simulink model "Uklad_simulink_vivado_trzy_sciezki_works"  (R2025b)
settings: Solver=VariableStepAuto  StartTime=0.0  StopTime=0.5  RelTol=1e-3
undefined symbols (not defined in the file or in its folder): c, dspblkCoreblockFVToolHelper, gcbh, sfvc784, xck26
libraries: hdlBasic x7, simulink x4, hdlDSPIP x3, hdlUtilities x2, vmcUtilities x1
settings Model: Creator=janek  LastModifiedBy=janek

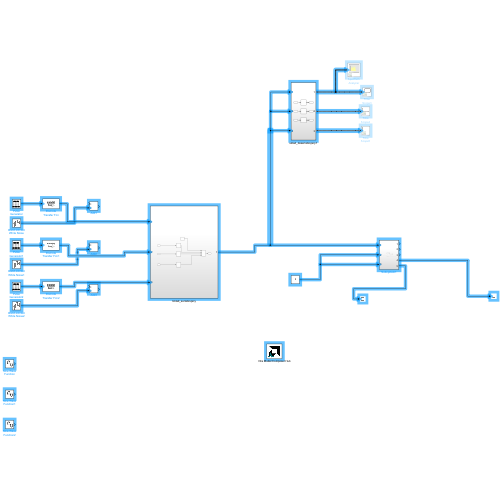
[thumbnail: Simulink's stored preview of the top-level diagram]
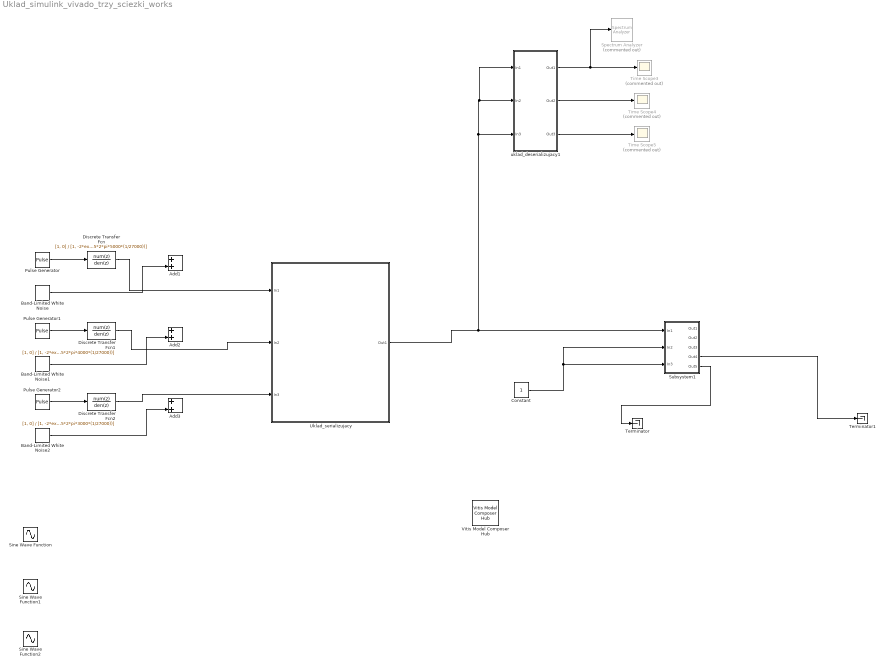
== system Uklad_simulink_vivado_trzy_sciezki_works ==
  Add1 : Sum
  Add2 : Sum
  Add3 : Sum
  Band-Limited White Noise : simulink/Sources/Band-Limited White Noise  Cov=[0.000001]  Ts=1/27000  seed=[23341]
  Band-Limited White Noise1 : simulink/Sources/Band-Limited White Noise  Cov=[0.000005]  Ts=1/27000  seed=[23341]
  Band-Limited White Noise2 : simulink/Sources/Band-Limited White Noise  Cov=[0.000005]  Ts=1/27000  seed=[23341]
  Constant : Constant
  Discrete Transfer Fcn : DiscreteTransferFcn  LoadFcn=dspblkCoreblockFVToolHelper(gcbh,'load');  Numerator=[1, 0]  Denominator=[1, -2*exp(-0.05*2*pi*5000*(1/27000))*cos(2*pi*5000*sqrt(1-0.05^2)*(1/27000)), exp(-2*0.05*2*pi*5000*(1/27000))]
      settings: CopyFcn=dspblkCoreblockFVToolHelper(gcbh,'copy');  DeleteFcn=dspblkCoreblockFVToolHelper(gcbh,'close');  ModelCloseFcn=dspblkCoreblockFVToolHelper(gcbh,'close');  PreSaveFcn=dspblkCoreblockFVToolHelper(gcbh,'presave');  PostSaveFcn=dspblkCoreblockFVToolHelper(gcbh,'postsave');  CloseFcn=dspblkCoreblockFVToolHelper(gcbh,'close');
  Discrete Transfer Fcn1 : DiscreteTransferFcn  LoadFcn=dspblkCoreblockFVToolHelper(gcbh,'load');  Numerator=[1, 0]  Denominator=[1, -2*exp(-0.05*2*pi*5000*(1/27000))*cos(2*pi*4000*sqrt(1-0.05^2)*(1/27000)), exp(-2*0.05*2*pi*4000*(1/27000))]
      settings: CopyFcn=dspblkCoreblockFVToolHelper(gcbh,'copy');  DeleteFcn=dspblkCoreblockFVToolHelper(gcbh,'close');  ModelCloseFcn=dspblkCoreblockFVToolHelper(gcbh,'close');  PreSaveFcn=dspblkCoreblockFVToolHelper(gcbh,'presave');  PostSaveFcn=dspblkCoreblockFVToolHelper(gcbh,'postsave');  CloseFcn=dspblkCoreblockFVToolHelper(gcbh,'close');
  Discrete Transfer Fcn2 : DiscreteTransferFcn  LoadFcn=dspblkCoreblockFVToolHelper(gcbh,'load');  Numerator=[1, 0]  Denominator=[1, -2*exp(-0.05*2*pi*5000*(1/27000))*cos(2*pi*3000*sqrt(1-0.05^2)*(1/27000)), exp(-2*0.05*2*pi*3000*(1/27000))]
      settings: CopyFcn=dspblkCoreblockFVToolHelper(gcbh,'copy');  DeleteFcn=dspblkCoreblockFVToolHelper(gcbh,'close');  ModelCloseFcn=dspblkCoreblockFVToolHelper(gcbh,'close');  PreSaveFcn=dspblkCoreblockFVToolHelper(gcbh,'presave');  PostSaveFcn=dspblkCoreblockFVToolHelper(gcbh,'postsave');  CloseFcn=dspblkCoreblockFVToolHelper(gcbh,'close');
  Pulse Generator : DiscretePulseGenerator  Period=540  SampleTime=1/27000
  Pulse Generator1 : DiscretePulseGenerator  Period=675  SampleTime=1/27000
  Pulse Generator2 : DiscretePulseGenerator  Period=900  SampleTime=1/27000
  Sine Wave Function : Sin  Frequency=2*pi*4000  SampleTime=1/27000
  Sine Wave Function1 : Sin  Frequency=2*pi*5000  SampleTime=1/27000
  Sine Wave Function2 : Sin  Frequency=2*pi*3000  SampleTime=1/27000
  Spectrum Analyzer : SpectrumAnalyzer  Commented=on  WindowPosition=[727.000000,50.000000,800.000000,510.000000,]  ScopeFrameLocation=window  SampleRateSource=Property  SampleRate=27000  WindowInvariantSamplesPerUpdate=on  Span=27000  StartFrequency=-13500  StopFrequency=13500  YLimits=[-62.2796 1.3485]  SelectedToolstripTab=spectrumAnalyzerToolstrip.measurementsTab
  Subsystem1 : Subsystem
  Terminator : Terminator
  Terminator1 : Terminator
  Time Scope3 : Scope  Commented=on
      settings: TimeUnits=Metric (based on Time Span)  ActiveDisplayYMinimum=-1.152524294390888  ActiveDisplayYMaximum=1.239169366043442  YLabel=Amplitude  DataLoggingVariableName=ScopeData6
  Time Scope4 : Scope  Commented=on
      settings: TimeUnits=Metric (based on Time Span)  ActiveDisplayYMinimum=-1.2987208316479313  ActiveDisplayYMaximum=1.398278565602173  YLabel=Amplitude  DataLoggingVariableName=ScopeData7
  Time Scope5 : Scope  Commented=on
      settings: TimeUnits=Metric (based on Time Span)  ActiveDisplayYMinimum=-1.5119749451959528  ActiveDisplayYMaximum=1.7752831879003923  YLabel=Amplitude  DataLoggingVariableName=ScopeData8
  Uklad_serializujacy : Subsystem
  Vitis Model Composer Hub : vmcUtilities/Vitis Model Composer Hub  Tag=genX  CodeGeneration=off  SubsystemName=Subsystem1  CompilationType=HDLCompilation  ExportTypeV2=IP Catalog  StartColumn=1  NumberOfColumns=1  TargetDirectory=./netlist  exportDesign=off  analyzeDesign=off  validateDesignOnHw=off  ExportType=AI Engines  IpVendor=xilinx.com  IpLibrary=hls  IpVersion=1.0  IpHWLanguage=Verilog  AieCompilerOptions={}  AieSimulatorOptions={}  CreateTestbench=off  TestbenchStackSize=10  RunRtlSim=off  RunCSim=off  RunAieSim=off  AieSimTimeout=50000  RunAieSimProfiling=off  LaunchVitisAnalyzer=off  PlotOutput=off  RunX86Sim=off  X86SimTimeout=10  GenHwImage=off  GenLibadfXo=on  GenHwValidationCode=off  PlatformType=Not Specified  HwSystemType=Baremetal  HwValidationTarget=hw  ProjDevice=Kria KR260 Robotics Starter Kit SOM (xck26-sfvc784-2LV-c)  ProjDevicePart=xck26-sfvc784-2LV-c  AIEType=None  SamplePeriod=-1  ClockFrequency=200  DataPathParallelism=1  xilinxfamily=zynquplus  part=xck26  speed=-2LV-c  package=sfvc784  directory=./netlist\ip\Subsystem1\src  testbench=off  incr_netlist=off  synthesis_tool=Vivado  clock_wrapper=Clock Enables  dbl_ovrd=According to Block Masks  dcm_input_clock_period=10  sysclk_period=1000  simulink_period=1/81000  eval_field=0  LogFileName=''  NThreads=4
  uklad_deserializujacy1 : Subsystem
  wires:
  Constant/1 -> Subsystem1/2(In2), Subsystem1/3(In3)
  Subsystem1/4(Out4) -> Terminator1/1
  Subsystem1/5(Out5) -> Terminator/1
  Uklad_serializujacy/1(Out1) -> uklad_deserializujacy1/1(In1), uklad_deserializujacy1/2(In2), uklad_deserializujacy1/3(In3), Subsystem1/1(In1)
  uklad_deserializujacy1/3(Out3) -> Time Scope5/1
  uklad_deserializujacy1/2(Out2) -> Time Scope4/1
  Pulse Generator/1 -> Discrete Transfer Fcn/1
  Band-Limited White Noise1/1 -> Add2/2
  Pulse Generator1/1 -> Discrete Transfer Fcn1/1
  Band-Limited White Noise2/1 -> Add3/2
  Pulse Generator2/1 -> Discrete Transfer Fcn2/1
  uklad_deserializujacy1/1(Out1) -> Spectrum Analyzer/1, Time Scope3/1
  Band-Limited White Noise/1 -> Add1/2
  Discrete Transfer Fcn/1 -> Uklad_serializujacy/1(In1)
  Discrete Transfer Fcn1/1 -> Uklad_serializujacy/2(In2)
  Discrete Transfer Fcn2/1 -> Uklad_serializujacy/3(In3)

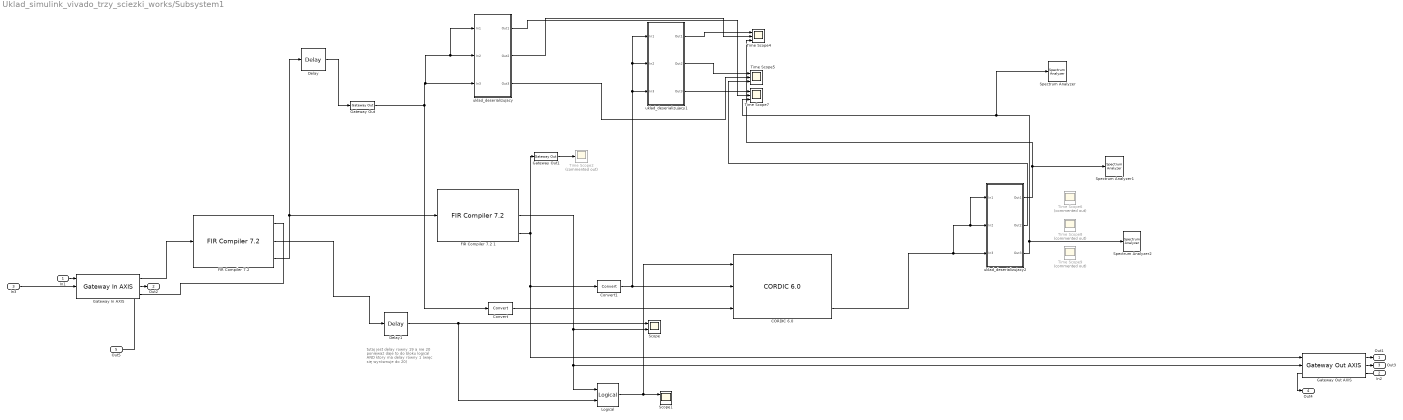
== system Uklad_simulink_vivado_trzy_sciezki_works/Subsystem1 ==
  note: tutaj jest delay rowny 19 a nie 20 ponieważ daje to do bloku logical AND ktory ma delay równy 1 (więc się wyrównuje do 20)
  In1 : Inport
  In2 : Inport  Port=2
  In3 : Inport  Port=3
  "CORDIC 6.0 " : hdlDSPIP/CORDIC 6.0   functional_selection=Translate  architectural_configuration=Parallel  pipelining_mode=Maximum  data_format=SignedFraction  phase_format=Radians  input_width=16  output_width=16  round_mode=Nearest_Even  iterations=0  precision=0  compensation_scaling=BRAM  coarse_rotation=on  aclken=off  aresetn=off  out_tready=off  cartesian_has_tuser=off  cartesian_has_tlast=off  cartesian_tuser_width=1  phase_has_tuser=off  phase_has_tlast=off  phase_tuser_width=1  out_tlast_behv=Null  flow_control=NonBlocking  optimize_goal=Resources  trim_axipin_name=on  simulation_type=hybrid_sim  simulation_model=sysgen:cordic_v6_0  data_path_portlist={'s_axis_cartesian_tdata_imag', 's_axis_cartesian_tdata_real', 's_axis_phase_tdata_phase', 'm_axis_dout_tdata_imag', 'm_axis_dout_tdata_real', 'm_axis_dout_tdata_phase','m_axis_dout_tdata'}  ip_name=CORDIC  ip_version=6.0  dsptool_ready=true  ipcore_usecache=true  ipcore_useipmodelcache=true  wrapper_available=true  port_translation_map={ 'aclken' => 'en', 'aresetn' => 'rst' }  XmcBlockStatus=1  maskContainerNames=group15  block_type=cordic_v6_0  block_config=sysgen:rodinimport_config  block_width=800
  Convert : hdlBasic/Convert  gui_display_data_type=Fixed-point  arith_type=Signed (2's comp)  n_bits=16  bin_pt=14  float_type=Single  exp_bits=8  fraction_bits=24  quantization="Round  (unbiased: +/- Inf)"  overflow=Wrap  en=off  latency=1  pipeline=off  XmcBlockStatus=1  maskContainerNames=group2  block_type=convert  block_config=sysgen:Convert_config  block_width=595  block_height=885
  Convert1 : hdlBasic/Convert  gui_display_data_type=Fixed-point  arith_type=Signed (2's comp)  n_bits=16  bin_pt=14  float_type=Single  exp_bits=8  fraction_bits=24  quantization="Round  (unbiased: +/- Inf)"  overflow=Saturate  en=off  latency=1  pipeline=off  XmcBlockStatus=1  maskContainerNames=group2  block_type=convert  block_config=sysgen:Convert_config  block_width=595  block_height=885
  Delay : hdlBasic/Delay  rst=off  en=off  latency=271  reg_retiming=off  XmcBlockStatus=1  maskContainerNames=group1  block_type=delay  block_config=sysgen:Delay_config
  Delay1 : hdlBasic/Delay  rst=off  en=off  latency=268  reg_retiming=off  XmcBlockStatus=1  maskContainerNames=group1  block_type=delay  block_config=sysgen:Delay_config
  "FIR Compiler 7.2 " : hdlDSPIP/FIR Compiler 7.2   coefficientvector=my_coefficients  coefficient_sets=1  coefficient_reload=off  filter_type=Single_Rate  rate_change_type=Integer  interpolation_rate=1  decimation_rate=1  zero_pack_factor=1  channel_sequence=Basic  number_channels=3  pattern_list='P4-0,P4-1,P4-2,P4-3,P4-4'  number_paths=1  ratespecification=Maximum_Possible  sampleperiod=1  hardwareoversamplingrate=1  coefficient_sign=Unsigned  quantization=Quantize_Only  coefficient_width=16  bestprecision=on  coefficient_fractional_bits=16  coefficient_structure=Inferred  output_rounding_mode=Convergent_Rounding_to_Even  output_width=16  filter_architecture=Systolic_Multiply_Accumulate  optimization_goal=Area  optimization_list='None'  data_buffer_type=Automatic  coefficient_buffer_type=Automatic  input_buffer_type=Automatic  output_buffer_type=Automatic  preference_for_other_storage=Automatic  multi_column_support=Automatic  columnconfig='46'  inter_column_pipe_length=4  data_has_tlast=Not_Required  m_data_has_tready=off  s_data_has_fifo=off  s_data_has_tuser=Not_Required  m_data_has_tuser=Not_Required  s_config_sync_mode=On_Vector  s_config_method=Single  num_reload_slots=1  has_aclken=off  has_aresetn=off  reset_data_vector=on  trim_axipin_name=on  simulation_type=hybrid_sim  simulation_model=sysgen:xfirv7_2_cmodel  data_path_portlist={ 's_axis_data_tdata', 'm_axis_data_tdata' }  passband_min=0.0  passband_max=0.5  stopband_min=0.5  stopband_max=1.0  filter_selection=1  gui_behaviour='Sysgen_GUI'  data_sign=Signed  data_width=16  data_fractional_bits=0  data_tuser_width=1  wrapper_available=true  ip_wrap_arbitrary_binary_point=true  ip_name=FIR Compiler  ip_version=7.2  dsptool_ready=true  ipcore_usecache=true  ipcore_useipmodelcache=true  port_translation_map={ 'aclken' => 'en', 'aresetn' => 'rst' }  run_core_at_system_period=true  ipcore_xco_need_fpga_part=true  ipcore_fpga_part=[]  XmcBlockStatus=1  maskContainerNames=tabcontainer1  block_type=fir_compiler_v7_2  block_config=sysgen:rodinimport_config  block_width=820  block_height=600
  FIR Compiler 7.2 1 : hdlDSPIP/FIR Compiler 7.2   coefficientvector=hilbert_coe  coefficient_sets=1  coefficient_reload=off  filter_type=Single_Rate  rate_change_type=Integer  interpolation_rate=1  decimation_rate=1  zero_pack_factor=1  channel_sequence=Basic  number_channels=3  pattern_list='P4-0,P4-1,P4-2,P4-3,P4-4'  number_paths=1  ratespecification=Maximum_Possible  sampleperiod=1  hardwareoversamplingrate=1  coefficient_sign=Unsigned  quantization=Quantize_Only  coefficient_width=16  bestprecision=on  coefficient_fractional_bits=15  coefficient_structure=Inferred  output_rounding_mode=Convergent_Rounding_to_Even  output_width=16  filter_architecture=Systolic_Multiply_Accumulate  optimization_goal=Area  optimization_list='None'  data_buffer_type=Automatic  coefficient_buffer_type=Automatic  input_buffer_type=Automatic  output_buffer_type=Automatic  preference_for_other_storage=Automatic  multi_column_support=Automatic  columnconfig='65'  inter_column_pipe_length=4  data_has_tlast=Not_Required  m_data_has_tready=off  s_data_has_fifo=off  s_data_has_tuser=Not_Required  m_data_has_tuser=Not_Required  s_config_sync_mode=On_Vector  s_config_method=Single  num_reload_slots=1  has_aclken=off  has_aresetn=off  reset_data_vector=on  trim_axipin_name=on  simulation_type=hybrid_sim  simulation_model=sysgen:xfirv7_2_cmodel  data_path_portlist={ 's_axis_data_tdata', 'm_axis_data_tdata' }  passband_min=0.0  passband_max=0.5  stopband_min=0.5  stopband_max=1.0  filter_selection=1  gui_behaviour='Sysgen_GUI'  data_sign=Signed  data_width=16  data_fractional_bits=0  data_tuser_width=1  wrapper_available=true  ip_wrap_arbitrary_binary_point=true  ip_name=FIR Compiler  ip_version=7.2  dsptool_ready=true  ipcore_usecache=true  ipcore_useipmodelcache=true  port_translation_map={ 'aclken' => 'en', 'aresetn' => 'rst' }  run_core_at_system_period=true  ipcore_xco_need_fpga_part=true  ipcore_fpga_part=[]  XmcBlockStatus=1  maskContainerNames=tabcontainer1  block_type=fir_compiler_v7_2  block_config=sysgen:rodinimport_config  block_width=820  block_height=600
  Gateway In AXIS : hdlUtilities/Gateway In AXIS  gui_display_data_type=Fixed-point  arith_type=Signed (2's comp)  n_bits=16  bin_pt=14  preci_type=Custom  exp_width=16  frac_width=24  quantization="Round  (unbiased: +/- Inf)"  overflow=Saturate  bool_to_boolean=off  OutSampleTime=1/81000  block_type=gatewayinaxi  XmcBlockStatus=1
  Gateway Out : hdlBasic/Gateway Out  inherit_from_input=off  bool_to_boolean=off  hdl_port=on  rows=1  columns=1  UseAsDAC=off  DACChannel='1'  interface=None  automatic_assignment=on  address_offset=hex2dec('00')  intf_name=''  intf_description=''  timing_constraint=None  locs_specified=off  LOCs={}  io_standard={}  XmcBlockStatus=1  maskContainerNames=group4  block_type=gatewayout  block_config=sysgen:gateway_out_config  block_width_w=590  block_height_w=620  block_width=620  block_height=750
  Gateway Out AXIS : hdlUtilities/Gateway Out AXIS  mask_sample_period=1/81000  bool_to_boolean=off  block_type=gatewayoutaxi
  Gateway Out1 : hdlBasic/Gateway Out  inherit_from_input=off  bool_to_boolean=off  hdl_port=on  rows=1  columns=1  UseAsDAC=off  DACChannel='1'  interface=None  automatic_assignment=on  address_offset=hex2dec('00')  intf_name=''  intf_description=''  timing_constraint=None  locs_specified=off  LOCs={}  io_standard={}  XmcBlockStatus=1  maskContainerNames=group4  block_type=gatewayout  block_config=sysgen:gateway_out_config  block_width_w=590  block_height_w=620  block_width=620  block_height=750
  Logical : hdlBasic/Logical  logical_function=AND  inputs=2  en=off  latency=1  precision=User Defined  arith_type=Boolean  n_bits=1  bin_pt=0  align_bp=on  overflow=[]  quantization=[]  XmcBlockStatus=1  maskContainerNames=tabcontainer1  block_type=logical  block_config=sysgen:Logical_config
  Scope : Scope  NumInputPorts=2
      settings: ActiveDisplayYMinimum=-0.12499999999999997  ActiveDisplayYMaximum=1.125  DataLoggingVariableName=ScopeData5
  Scope1 : Scope  NumInputPorts=2
      settings: ActiveDisplayYMinimum=0.47844827586206895  ActiveDisplayYMaximum=0.53722570532915359  DataLoggingVariableName=ScopeData3
  Spectrum Analyzer : SpectrumAnalyzer  WindowPosition=[617.000000,1935.000000,800.000000,500.000000,]  Visible=on  ScopeFrameLocation=window  SampleRateSource=Property  SampleRate=27000  WindowInvariantSamplesPerUpdate=on  Span=27000  StartFrequency=-13500  StopFrequency=13500  YLimits=[-51.8942 11.6038]  SelectedToolstripTab=spectrumAnalyzerToolstrip.measurementsTab
  Spectrum Analyzer1 : SpectrumAnalyzer  WindowPosition=[594.000000,1624.000000,800.000000,500.000000,]  Visible=on  ScopeFrameLocation=window  SampleRateSource=Property  SampleRate=27000  WindowInvariantSamplesPerUpdate=on  Span=27000  StartFrequency=-13500  StopFrequency=13500  YLimits=[-56.0285 10.5734]  SelectedToolstripTab=spectrumAnalyzerToolstrip.measurementsTab
  Spectrum Analyzer2 : SpectrumAnalyzer  WindowPosition=[590.000000,1323.000000,800.000000,500.000000,]  Visible=on  ScopeFrameLocation=window  SampleRateSource=Property  SampleRate=27000  WindowInvariantSamplesPerUpdate=on  Span=27000  StartFrequency=-13500  StopFrequency=13500  YLimits=[-51.8031 11.7152]  SelectedToolstripTab=spectrumAnalyzerToolstrip.measurementsTab
  Time Scope{2,6,8..9} (4 alike) : Scope  Commented=on
      Time Scope2 settings: TimeUnits=Metric (based on Time Span)  ActiveDisplayYMinimum=-1.2635498046875  ActiveDisplayYMaximum=1.2645263671875  YLabel=Amplitude  DataLoggingVariableName=ScopeData9
      Time Scope6 settings: TimeUnits=Metric (based on Time Span)  ActiveDisplayYMinimum=-0.15950012207031247  ActiveDisplayYMaximum=1.4355010986328125  YLabel=Amplitude  DataLoggingVariableName=ScopeData11
      Time Scope8 settings: TimeUnits=Metric (based on Time Span)  ActiveDisplayYMinimum=-0.19171905517578119  ActiveDisplayYMaximum=1.7254714965820312  YLabel=Amplitude  DataLoggingVariableName=ScopeData12
      Time Scope9 settings: TimeUnits=Metric (based on Time Span)  ActiveDisplayYMinimum=-0.12494659423828122  ActiveDisplayYMaximum=1.1245193481445312  YLabel=Amplitude  DataLoggingVariableName=ScopeData13
  Time Scope4 : Scope  NumInputPorts=3
      settings: TimeUnits=Metric (based on Time Span)  ActiveDisplayYMinimum=-1.2568082493662045  ActiveDisplayYMaximum=1.6676912623525455  YLabel=Amplitude
  Time Scope5 : Scope  NumInputPorts=3
      settings: TimeUnits=Metric (based on Time Span)  ActiveDisplayYMinimum=-1.3144606578199167  ActiveDisplayYMaximum=1.7754441273363333  YLabel=Amplitude
  Time Scope7 : Scope  NumInputPorts=3
      settings: TimeUnits=Metric (based on Time Span)  ActiveDisplayYMinimum=-1.2389688612539558  ActiveDisplayYMaximum=1.7163534043710442  YLabel=Amplitude  DataLoggingVariableName=ScopeData2
  uklad_deserializujacy : Subsystem
  uklad_deserializujacy1 : Subsystem
  uklad_deserializujacy2 : Subsystem
  Out1 : Outport
  Out2 : Outport  Port=2
  Out3 : Outport  Port=3
  Out4 : Outport  Port=4
  Out5 : Outport  Port=5
  wires:
  Gateway In AXIS/3 -> Out5/1
  In3/1 -> Gateway In AXIS/2
  In2/1 -> Gateway Out AXIS/3
  Gateway Out AXIS/1 -> Out1/1
  Gateway Out AXIS/3 -> Out4/1
  In1/1 -> Gateway In AXIS/1
  Gateway Out AXIS/2 -> Out3/1
  Gateway In AXIS/2 -> Out2/1
  Gateway In AXIS/1 -> "FIR Compiler 7.2 "/1
  "FIR Compiler 7.2 "/1 -> Gateway In AXIS/3
  FIR Compiler 7.2 1/3 -> Gateway Out1/1, Convert1/1, Gateway Out AXIS/1
  uklad_deserializujacy1/2(Out2) -> Time Scope5/1
  uklad_deserializujacy1/1(Out1) -> Time Scope4/1
  uklad_deserializujacy1/3(Out3) -> Time Scope7/1
  "FIR Compiler 7.2 "/3 -> Delay/1, FIR Compiler 7.2 1/1
  Delay/1 -> Gateway Out/1
  Gateway Out1/1 -> Time Scope2/1
  FIR Compiler 7.2 1/2 -> Logical/1, Gateway Out AXIS/2, Scope/2
  "FIR Compiler 7.2 "/2 -> Delay1/1
  Delay1/1 -> Logical/2, Scope/1
  Logical/1 -> "CORDIC 6.0 "/1, Scope1/1
  Convert/1 -> "CORDIC 6.0 "/3
  Convert1/1 -> uklad_deserializujacy1/1(In1), uklad_deserializujacy1/2(In2), uklad_deserializujacy1/3(In3), "CORDIC 6.0 "/2
  uklad_deserializujacy/1(Out1) -> Time Scope7/2
  uklad_deserializujacy/2(Out2) -> Time Scope4/2
  uklad_deserializujacy/3(Out3) -> Time Scope5/2
  uklad_deserializujacy2/1(Out1) -> Time Scope4/3, Spectrum Analyzer1/1
  uklad_deserializujacy2/2(Out2) -> Time Scope5/3
  uklad_deserializujacy2/3(Out3) -> Spectrum Analyzer2/1, Spectrum Analyzer/1, Time Scope7/3
  "CORDIC 6.0 "/3 -> uklad_deserializujacy2/1(In1), uklad_deserializujacy2/2(In2), uklad_deserializujacy2/3(In3)
  Gateway Out/1 -> Convert/1, uklad_deserializujacy/1(In1), uklad_deserializujacy/2(In2), uklad_deserializujacy/3(In3)

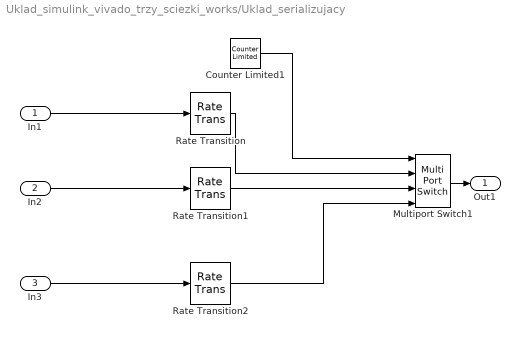
== system Uklad_simulink_vivado_trzy_sciezki_works/Uklad_serializujacy ==
  In1 : Inport
  In2 : Inport  Port=2
  In3 : Inport  Port=3
  Counter Limited1 : simulink/Sources/Counter Limited  uplimit=2  tsamp=1/81000
  Multiport Switch1 : MultiPortSwitch  DataPortOrder=Zero-based contiguous  zeroidx=on  SaturateOnIntegerOverflow=off  InputSameDT=off
  Rate Transition : RateTransition  OutPortSampleTime=1/81000
  Rate Transition1 : RateTransition  OutPortSampleTime=1/81000
  Rate Transition2 : RateTransition  OutPortSampleTime=1/81000
  Out1 : Outport
  wires:
  In1/1 -> Rate Transition/1
  Rate Transition2/1 -> Multiport Switch1/4
  Counter Limited1/1 -> Multiport Switch1/1
  Rate Transition1/1 -> Multiport Switch1/3
  In2/1 -> Rate Transition1/1
  Rate Transition/1 -> Multiport Switch1/2
  In3/1 -> Rate Transition2/1
  Multiport Switch1/1 -> Out1/1

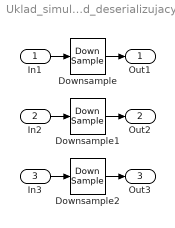
== system Uklad_simulink_vivado_trzy_sciezki_works/uklad_deserializujacy1 ==
  In1 : Inport
  In2 : Inport  Port=2
  In3 : Inport  Port=3
  Downsample : DownSample  N=3  AllowArbitraryFixedInput=on
  Downsample1 : DownSample  N=3  phase=1  AllowArbitraryFixedInput=on
  Downsample2 : DownSample  N=3  phase=2  AllowArbitraryFixedInput=on
  Out1 : Outport
  Out2 : Outport  Port=2
  Out3 : Outport  Port=3
  wires:
  In3/1 -> Downsample2/1
  In1/1 -> Downsample/1
  Downsample/1 -> Out1/1
  In2/1 -> Downsample1/1
  Downsample2/1 -> Out3/1
  Downsample1/1 -> Out2/1

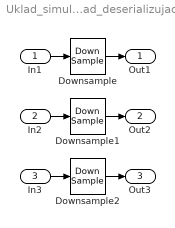
== system Uklad_simulink_vivado_trzy_sciezki_works/Subsystem1/uklad_deserializujacy ==
  In1 : Inport
  In2 : Inport  Port=2
  In3 : Inport  Port=3
  Downsample : DownSample  N=3  AllowArbitraryFixedInput=on
  Downsample1 : DownSample  N=3  phase=1  AllowArbitraryFixedInput=on
  Downsample2 : DownSample  N=3  phase=2  AllowArbitraryFixedInput=on
  Out1 : Outport
  Out2 : Outport  Port=2
  Out3 : Outport  Port=3
  wires:
  In3/1 -> Downsample2/1
  In1/1 -> Downsample/1
  Downsample/1 -> Out1/1
  In2/1 -> Downsample1/1
  Downsample2/1 -> Out3/1
  Downsample1/1 -> Out2/1

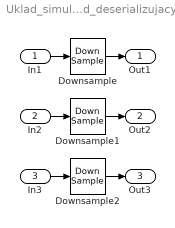
== system Uklad_simulink_vivado_trzy_sciezki_works/Subsystem1/uklad_deserializujacy1 ==
  In1 : Inport
  In2 : Inport  Port=2
  In3 : Inport  Port=3
  Downsample : DownSample  N=3  AllowArbitraryFixedInput=on
  Downsample1 : DownSample  N=3  phase=1  AllowArbitraryFixedInput=on
  Downsample2 : DownSample  N=3  phase=2  AllowArbitraryFixedInput=on
  Out1 : Outport
  Out2 : Outport  Port=2
  Out3 : Outport  Port=3
  wires:
  In3/1 -> Downsample2/1
  In1/1 -> Downsample/1
  Downsample/1 -> Out1/1
  In2/1 -> Downsample1/1
  Downsample2/1 -> Out3/1
  Downsample1/1 -> Out2/1

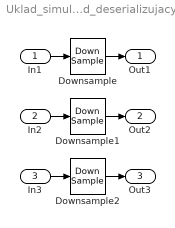
== system Uklad_simulink_vivado_trzy_sciezki_works/Subsystem1/uklad_deserializujacy2 ==
  In1 : Inport
  In2 : Inport  Port=2
  In3 : Inport  Port=3
  Downsample : DownSample  N=3  AllowArbitraryFixedInput=on
  Downsample1 : DownSample  N=3  phase=1  AllowArbitraryFixedInput=on
  Downsample2 : DownSample  N=3  phase=2  AllowArbitraryFixedInput=on
  Out1 : Outport
  Out2 : Outport  Port=2
  Out3 : Outport  Port=3
  wires:
  In3/1 -> Downsample2/1
  In1/1 -> Downsample/1
  Downsample/1 -> Out1/1
  In2/1 -> Downsample1/1
  Downsample2/1 -> Out3/1
  Downsample1/1 -> Out2/1
